simulink model "SPNF2"  (R2022a)
settings: Solver=FixedStepDiscrete  StartTime=0.0  StopTime=xin.TimeInfo.End  RelTol=1e-3
values from neighbouring files (symbols this model uses):
  Ts = 1e-6    (= 1e-06)    [NLD1sim.m]    (also in NLD2sim.m; SPNF1sim.m; SPNF2sim.m)
undefined symbols (not defined in the file or in its folder): cols
settings Model: Creator=dileepan  LastModifiedBy=dileepan
settings SolverCC: AlgebraicLoopSolver=TrustRegion
settings DataIOCC: SaveFormat=Array  SaveOutput=off  SignalLogging=off  DSMLogging=off  SaveTime=off  ReturnWorkspaceOutputs=off
settings DebuggingCC: UnconnectedInputMsg=warning  UnconnectedOutputMsg=warning  UnconnectedLineMsg=warning  SFMachineParentedDataDiag=warning
settings RTWCC: DLArmComputeVersion=19.05

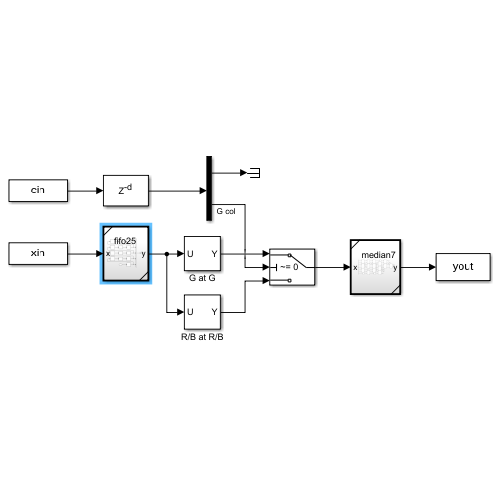
[thumbnail: Simulink's stored preview of the top-level diagram]
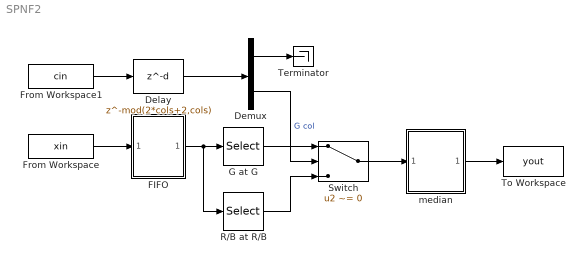
== system SPNF2 ==
  Delay : Delay  DelayLength=mod(2*cols+2,cols)
  Demux : Demux  Outputs=2
  FIFO : Subsystem  TreatAsAtomicUnit=on  ReferencedSubsystem=fifo25
  From Workspace : FromWorkspace  VariableName=xin  SampleTime=Ts
  From Workspace1 : FromWorkspace  VariableName=cin  SampleTime=Ts
  G at G : Selector  InputPortWidth=25  IndexOptions=Index vector (dialog)  Indices=[7 9 13 13 13 17 19]  OutputSizes=1
  R/B at R/B : Selector  InputPortWidth=25  IndexOptions=Index vector (dialog)  Indices=[3 11 13 13 13 15 23]  OutputSizes=1
  Switch : Switch  Criteria=u2 ~= 0  SaturateOnIntegerOverflow=off  InputSameDT=off
  Terminator : Terminator
  To Workspace : ToWorkspace  VariableName=yout  SaveFormat=Timeseries  SampleTime=-1
  median : Subsystem  TreatAsAtomicUnit=on  ReferencedSubsystem=median7
  wires:
  Demux/2 -> Switch/2  "G col"
  Demux/1 -> Terminator/1
  median/1 -> To Workspace/1
  Switch/1 -> median/1
  From Workspace1/1 -> Delay/1
  G at G/1 -> Switch/1
  Delay/1 -> Demux/1
  R/B at R/B/1 -> Switch/3
  From Workspace/1 -> FIFO/1
  FIFO/1 -> R/B at R/B/1, G at G/1
